simulink model "cruisecontrol"  (R2020b)
settings: Solver=VariableStepAuto  StartTime=0.0  StopTime=10.0  RelTol=1e-3
values from neighbouring files (symbols this model uses):
  b = 50    [parameters.m]
  m = 1000    [parameters.m]
settings Model: Creator=sushma  LastModifiedBy=sushma

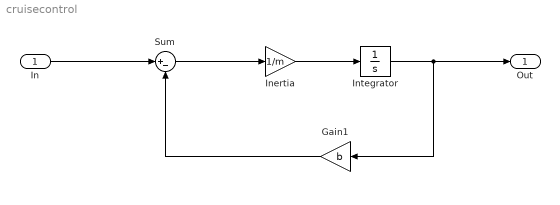
== system cruisecontrol ==
  In : Inport
  Gain1 : Gain  Gain=b
  Inertia : Gain  Gain=1/m
  Integrator : Integrator
  Sum : Sum  Inputs=|+-
  Out : Outport
  wires:
  Inertia/1 -> Integrator/1
  In/1 -> Sum/1
  Sum/1 -> Inertia/1
  Gain1/1 -> Sum/2
  Integrator/1 -> Gain1/1, Out/1
